simulink model "icl_control_sim_io"  (R2021a)
settings: Solver=FixedStepAuto  StartTime=0.0  StopTime=inf  FixedStep=Ts  RelTol=1e-3  EnableMultiTasking=on
InitFcn:
  | Ts = 0.001; % sample time
  | Tc = 0.008; % controller sample time
settings Model: SimulationMode=external  ExtModeEnableFloating=off  ExplicitPartitioning=on  Creator=zhaoyx  LastModifiedBy=Charles
settings SolverCC: ConcurrentTasks=on  AlgebraicLoopSolver=TrustRegion  PositivePriorityOrder=on  AutoInsertRateTranBlk=on  InsertRTBMode=Never (minimum delay)
settings DataIOCC: SaveFormat=StructureWithTime  ReturnWorkspaceOutputs=off
settings OptimizationCC: BlockReduction=off  DefaultParameterBehavior=Inlined  OptimizeBlockIOStorage=off  BufferReuse=off  GlobalBufferReuse=off  ExpressionFolding=off  LocalBlockOutputs=off  OptimizeDataStoreBuffers=off  BusAssignmentInplaceUpdate=off
settings DebuggingCC: TasksWithSamePriorityMsg=none  SFMachineParentedDataDiag=warning  ArithmeticOperatorsInVariantConditions=warning
settings HardwareCC: ProdBitPerLong=64  ProdLongLongMode=on  ProdHWDeviceType=Intel->x86-64 (Linux 64)
settings SFSimCC: CustomCodeUndefinedFunction=UseInterfaceOnly
settings RTWCC: Description=Simulink Real-Time  SystemTargetFile=slrealtime.tlc  TemplateMakefile=slrealtime_default_tmf  Toolchain=Simulink Real-Time Toolchain  BuildConfiguration=Faster Runs  CodeExecutionProfiling=on  TargetLang=C++
settings CodeAppCC: MaxIdLength=95

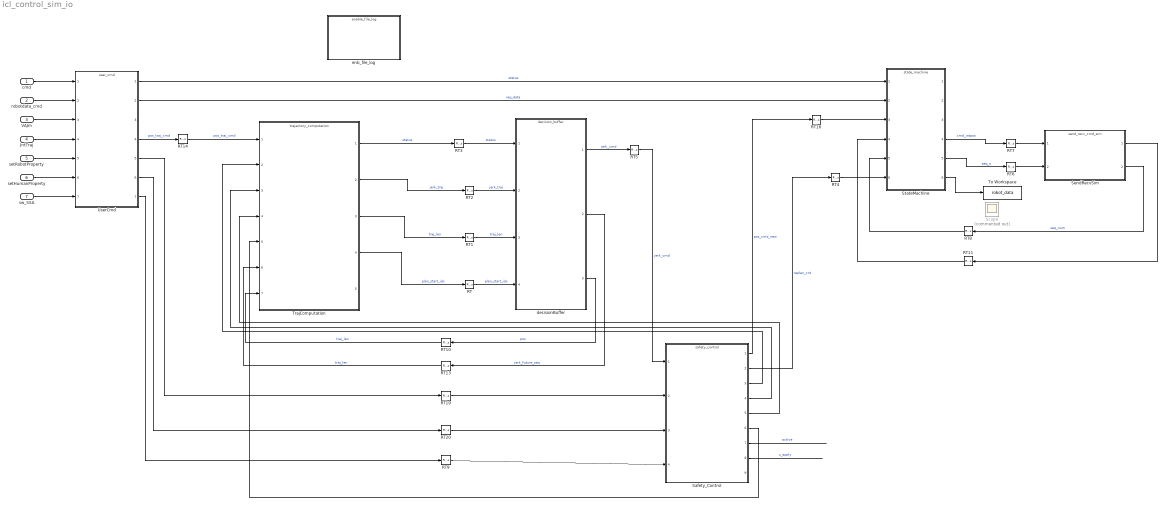
== system icl_control_sim_io ==
  cmd : Inport
  robotdata_cmd : Inport  Port=2
  VAJm : Inport  Port=3
  JntTraj : Inport  Port=4
  setRobotProperty : Inport  Port=5
  setHumanProperty : Inport  Port=6
  sw_SSA : Inport  Port=7
  RT{,1..3,6..10,13,19..20} (12 alike) : RateTransition  Deterministic=off
  RT11 : RateTransition  Deterministic=off  OutPortSampleTime=0.001
  RT14 : RateTransition  Deterministic=off  OutPortSampleTime=0.008
  RT16 : RateTransition  Deterministic=off  OutPortSampleTime=0.001
  RT4 : RateTransition  Deterministic=off  OutPortSampleTime=0.001
  RT5 : RateTransition  Deterministic=off  OutPortSampleTime=0.008
  Safety_Control : ModelReference  ModelNameDialog=safety_control.slx  SimulationMode=Normal  ModelReferenceVersion=1.580
  Scope : Scope  Commented=on
  SendRecvSim : ModelReference  ModelNameDialog=send_recv_cmd_sim.slx  SimulationMode=Normal  ModelReferenceVersion=1.66
  StateMachine : ModelReference  ModelNameDialog=state_machine.slx  SimulationMode=Normal  ModelReferenceVersion=1.108
  To Workspace : ToWorkspace  VariableName=robot_data  SampleTime=-1
  TrajComputation : ModelReference  ModelNameDialog=trajectory_computation.slx  SimulationMode=Normal  ModelReferenceVersion=1.226
  UserCmd : ModelReference  ModelNameDialog=user_cmd.slx  SimulationMode=Normal  ModelReferenceVersion=1.58
  decisionBuffer : ModelReference  ModelNameDialog=decision_buffer.slx  SimulationMode=Normal  ModelReferenceVersion=1.204
  enb_file_log : ModelReference  ModelNameDialog=enable_file_log.slx  SimulationMode=Normal  ModelReferenceVersion=1.2
  wires:
  StateMachine/4 -> RT7/1  "cmd_jntpos"
  StateMachine/5 -> RT6/1  "seq_o"
  UserCmd/1 -> StateMachine/1  "status"
  UserCmd/2 -> StateMachine/2  "req_data"
  SendRecvSim/2 -> RT8/1  "seq_num"
  TrajComputation/1 -> RT3/1  "status"
  decisionBuffer/1 -> RT5/1  "jerk_cmd"
  TrajComputation/2 -> RT2/1  "jerk_traj"
  TrajComputation/3 -> RT1/1  "traj_len"
  TrajComputation/4 -> RT/1  "plan_start_idx"
  UserCmd/4 -> RT14/1  "pos_traj_cmd"
  decisionBuffer/3 -> RT10/1  "pos"
  RT/1 -> decisionBuffer/4  "plan_start_idx"
  RT1/1 -> decisionBuffer/3  "traj_len"
  RT2/1 -> decisionBuffer/2  "jerk_traj"
  RT3/1 -> decisionBuffer/1  "status"
  RT6/1 -> SendRecvSim/2
  RT7/1 -> SendRecvSim/1
  RT8/1 -> StateMachine/5
  RT10/1 -> TrajComputation/7  "traj_len"
  RT13/1 -> TrajComputation/6  "traj_len"
  RT14/1 -> TrajComputation/1  "pos_traj_cmd"
  UserCmd/6 -> RT20/1
  decisionBuffer/2 -> RT13/1  "jerk_future_seq"
  UserCmd/5 -> RT19/1
  Safety_Control/1 -> RT16/1  "pos_cmd_new"
  RT16/1 -> StateMachine/3
  Safety_Control/2 -> RT4/1  "replan_cnt"
  RT19/1 -> Safety_Control/2
  RT20/1 -> Safety_Control/3
  Safety_Control/4 -> TrajComputation/3
  Safety_Control/3 -> TrajComputation/2
  RT4/1 -> StateMachine/6
  Safety_Control/6 -> TrajComputation/5
  RT5/1 -> Safety_Control/1  "jerk_cmd"
  Safety_Control/5 -> TrajComputation/4
  SendRecvSim/1 -> RT11/1
  RT11/1 -> StateMachine/4
  UserCmd/7 -> RT9/1
  RT9/1 -> Safety_Control/4
  Safety_Control/7 -> ?  "active"
  Safety_Control/8 -> ?  "u_apply"
  StateMachine/6 -> To Workspace/1
  cmd/1 -> UserCmd/1
  robotdata_cmd/1 -> UserCmd/2
  VAJm/1 -> UserCmd/3
  JntTraj/1 -> UserCmd/4
  setRobotProperty/1 -> UserCmd/5
  setHumanProperty/1 -> UserCmd/6
  sw_SSA/1 -> UserCmd/7
